simulink model "oltf"  (R2025b)
settings: Solver=VariableStepAuto  StartTime=0.0  StopTime=10.0  RelTol=1e-3
values from neighbouring files (symbols this model uses):
  den_ac = den_ac_1    [rlelog6.m]
  Kp = Kp_ac_1    (= 3.5)    [rlelog6.m]
  num_ac = num_ac_1    [rlelog6.m]
  R = 0.725    [rlelog6.m]
settings Model: Creator=t0900  LastModifiedBy=t0900

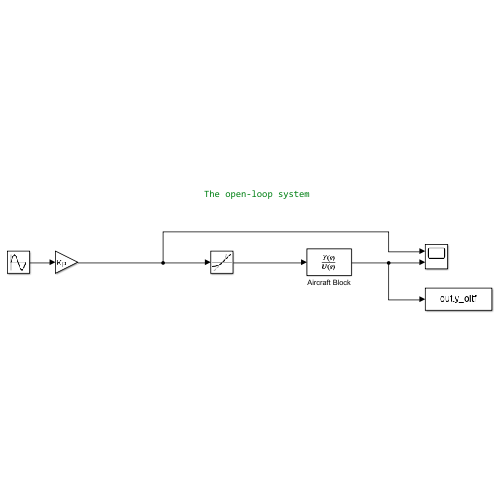
[thumbnail: Simulink's stored preview of the top-level diagram]
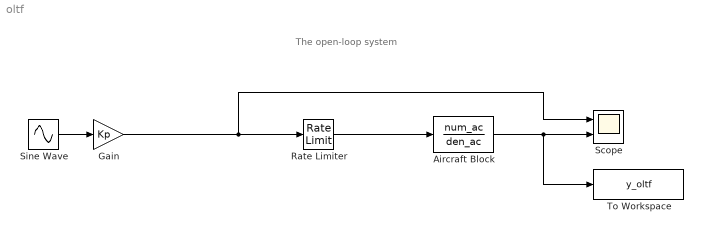
== system oltf ==
  note: The open-loop system
  Aircraft Block : TransferFcn  Numerator=num_ac  Denominator=den_ac
  Gain : Gain  Gain=Kp
  Rate Limiter : RateLimiter  RisingSlewLimit=R  FallingSlewLimit=-R
  Scope : Scope  NumInputPorts=2
      settings: ActiveDisplayYMinimum=-0.37468698741779388  ActiveDisplayYMaximum=3.404602506157413  YLabel=Pilot Command
  Sine Wave : Sin  SampleTime=0
  To Workspace : ToWorkspace  VariableName=y_oltf  SaveFormat=Timeseries  SampleTime=-1
  wires:
  Gain/1 -> Rate Limiter/1, Scope/1
  Rate Limiter/1 -> Aircraft Block/1
  Aircraft Block/1 -> To Workspace/1, Scope/2
  Sine Wave/1 -> Gain/1
